simulink model "M4_VehicleDynamics"  (R2026a)
settings: Solver=ode3  FixedStep=0.1
PreLoadFcn:
  | createM4BusObjects
undefined symbols (not defined in the file or in its folder): x0
settings Model: Creator=jeevan  LastModifiedBy=jeevan

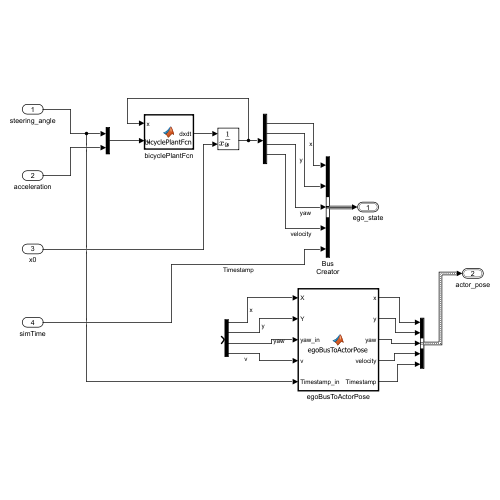
[thumbnail: Simulink's stored preview of the top-level diagram]
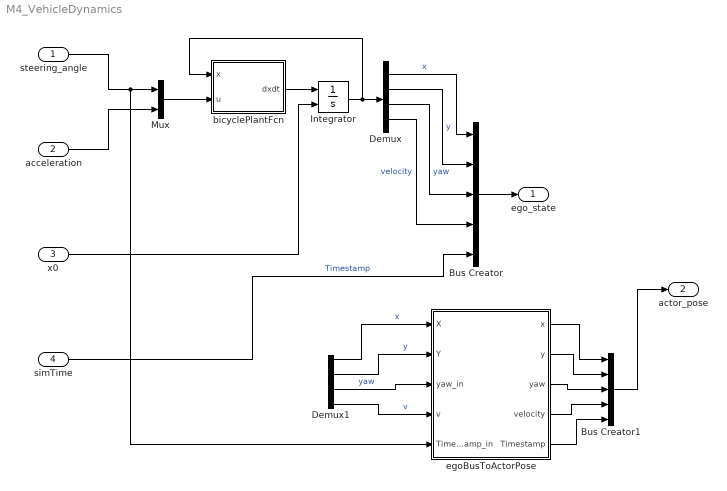
== system M4_VehicleDynamics ==
  steering_angle : Inport  OutDataTypeStr=double
  acceleration : Inport  Port=2  OutDataTypeStr=double
  x0 : Inport  Port=3  OutDataTypeStr=double  PortDimensions=4
  simTime : Inport  Port=4  OutDataTypeStr=double
  Bus Creator : BusCreator  Inputs=5  OutDataTypeStr=Bus: SihEgoBus
  Bus Creator1 : BusCreator  Inputs=5  OutDataTypeStr=Bus: SihEgoBus  NonVirtualBus=on
  Demux : Demux
  Demux1 : Demux
  Integrator : Integrator  InitialConditionSource=external  InitialCondition=x0
  Mux : Mux  Inputs=2
  bicyclePlantFcn : MATLAB Function  TreatAsAtomicUnit=on
  egoBusToActorPose : MATLAB Function  TreatAsAtomicUnit=on
  ego_state : Outport  OutDataTypeStr=Bus: SihEgoBus  BusOutputAsStruct=on
  actor_pose : Outport  Port=2  OutDataTypeStr=Bus: SihEgoBus  BusOutputAsStruct=on
  wires:
  x0/1 -> Integrator/2
  bicyclePlantFcn/1(dxdt) -> Integrator/1
  Mux/1 -> bicyclePlantFcn/2(u)
  steering_angle/1 -> Mux/1, egoBusToActorPose/5(Timestamp_in)
  acceleration/1 -> Mux/2
  Integrator/1 -> bicyclePlantFcn/1(x), Demux/1
  Bus Creator/1 -> ego_state/1
  Demux/1 -> Bus Creator/1  "x"
  Demux/2 -> Bus Creator/2  "y"
  Demux/3 -> Bus Creator/3  "yaw"
  Demux/4 -> Bus Creator/4  "velocity"
  simTime/1 -> Bus Creator/5  "Timestamp"
  Demux1/1 -> egoBusToActorPose/1(X)  "x"
  Demux1/2 -> egoBusToActorPose/2(Y)  "y"
  Demux1/3 -> egoBusToActorPose/3(yaw_in)  "yaw"
  Demux1/4 -> egoBusToActorPose/4(v)  "v"
  egoBusToActorPose/1(x) -> Bus Creator1/1
  egoBusToActorPose/2(y) -> Bus Creator1/2
  egoBusToActorPose/3(yaw) -> Bus Creator1/3
  egoBusToActorPose/4(velocity) -> Bus Creator1/4
  egoBusToActorPose/5(Timestamp) -> Bus Creator1/5
  Bus Creator1/1 -> actor_pose/1

== matlab function M4_VehicleDynamics/egoBusToActorPose ==
  data: X input; x output; Y input; yaw_in input; v input; Timestamp_in input; y output; yaw output; velocity output; Timestamp output
function [x, y, yaw, velocity, Timestamp] = egoBusToActorPose(X, Y, yaw_in, v, Timestamp_in)
%#codegen

x = X;
y = Y;
yaw = yaw_in;
velocity = v;
Timestamp = Timestamp_in;

== matlab function M4_VehicleDynamics/bicyclePlantFcn ==
  data: x input; u input; dxdt output
function dxdt = bicyclePlantFcn(x, u)
%#codegen

L = 2.5;

dxdt = [ x(4)*cos(x(3));
         x(4)*sin(x(3));
         x(4)/L*tan(u(1));
         u(2) ];
